simulink model "FIR_Filter"  (R2020b)
settings: Solver=VariableStepAuto  StartTime=0.0  StopTime=10.0  RelTol=1e-3
model workspace (MAT data in the model file):
  a1 = 2
  a2 = -3
  a3 = -4
  a4 = 5
settings Model: Creator=user  LastModifiedBy=user
settings DataIOCC: SaveOutput=off  SaveTime=off

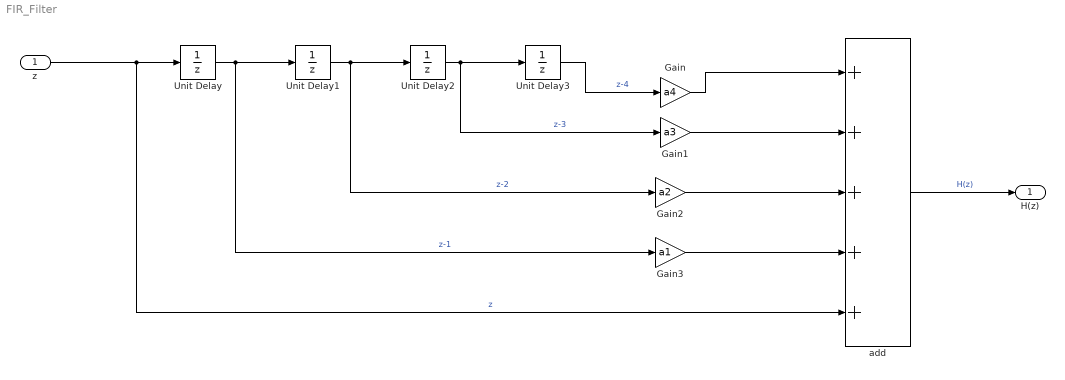
== system FIR_Filter ==
  z : Inport  OutDataTypeStr=double  PortDimensions=1  SampleTime=0
  Gain : Gain  Gain=a4
  Gain1 : Gain  Gain=a3
  Gain2 : Gain  Gain=a2
  Gain3 : Gain  Gain=a1
  Unit Delay{,1..3} (4 alike) : UnitDelay  SampleTime=-1  HasFrameUpgradeWarning=on
  add : Sum  Inputs=+++++
  H(z) : Outport  OutDataTypeStr=double  PortDimensions=1  SampleTime=0
  wires:
  Gain3/1 -> add/4
  z/1 -> Unit Delay/1, add/5  "z"
  Gain/1 -> add/1
  Gain1/1 -> add/2
  Unit Delay1/1 -> Unit Delay2/1, Gain2/1  "z-2"
  Unit Delay2/1 -> Unit Delay3/1, Gain1/1  "z-3"
  Gain2/1 -> add/3
  Unit Delay/1 -> Unit Delay1/1, Gain3/1  "z-1"
  Unit Delay3/1 -> Gain/1  "z-4"
  add/1 -> H(z)/1  "H(z)"
